simulink model "Nonlinear_Simulink"  (R2025b)
settings: Solver=VariableStepAuto  StartTime=0.0  StopTime=10.0  RelTol=1e-3
undefined symbols (not defined in the file or in its folder): p
settings Model: Creator=chako  LastModifiedBy=emma

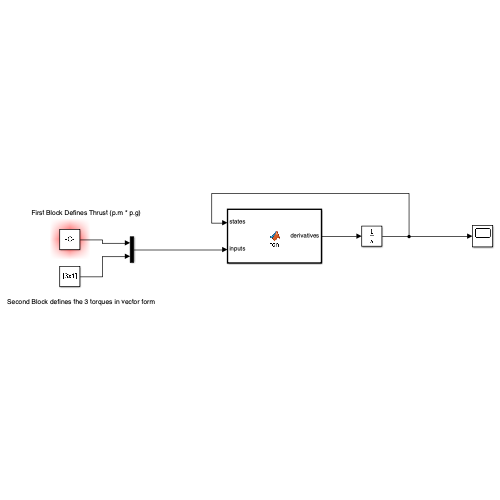
[thumbnail: Simulink's stored preview of the top-level diagram]
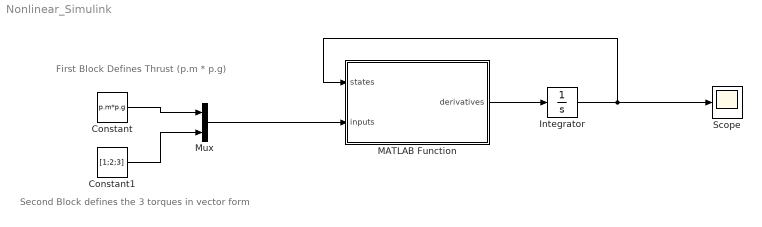
== system Nonlinear_Simulink ==
  note: First Block Defines Thrust (p.m * p.g)
  note: Second Block defines the 3 torques in vector form
  Constant : Constant  Value=p.m*p.g
  Constant1 : Constant  Value=[1;2;3]
  Integrator : Integrator
  MATLAB Function : MATLAB Function  TreatAsAtomicUnit=on
  Mux : Mux  Inputs=2
  Scope : Scope
  wires:
  MATLAB Function/1(derivatives) -> Integrator/1
  Integrator/1 -> MATLAB Function/1(states), Scope/1
  Mux/1 -> MATLAB Function/2(inputs)
  Constant/1 -> Mux/1
  Constant1/1 -> Mux/2

== matlab function Nonlinear_Simulink/MATLAB Function ==
  data: states input size=12; derivatives output size=12; inputs input size=4; parameters parameter
function derivatives = fcn(states, inputs, parameters)

 % I is the inertia matrix
    I = [p.Ixx 0 0;
         0 p.Iyy 0;
         0 0 p.Izz];

    xi= states(1:3); % x, y, z
    xid = states(4:6); %x_prime, y_prime, z_prime
    eta = states(7:9); % roll, pitch, yaw
    etad = states(10:12); % roll_prime, pitch_prime, yaw_prime

    % Cosines of each
    c_roll = cos(eta(1));
    c_pitch = cos(eta(2));
    c_yaw = cos(eta(3));

    % Sines of each
    s_roll = sin(eta(1));
    s_pitch = sin(eta(2));
    s_yaw = sin(eta(3));


    % Derivative of xi is xid

    % Calculative derivatives of xid
    xidd = [0;0;-p.g] - (p.kD/p.m)*xid + ...
        [s_roll*s_yaw + c_roll*s_pitch*c_yaw;
         c_roll*s_pitch*s_yaw - s_roll*c_yaw;
         c_roll*c_pitch]*inputs(1);


    % Derivative of eta is etad
    % Calculative derivatives of etad


    % eta is [phi, theta, psi] = roll pitch yaw
    W = [1  0       -s_pitch;
         0  c_roll  s_phi * c_pitch;
         0 -s_roll  c_roll * c_pitch];
    % v is rpy in body frame
    
    tau_body = [inputs(2);
                inputs(3);
                inputs(4)];
    v = W * etad;
    vd = inv(I) * (tau_body + [(p.Iyy - Izz)*v(2)*v(3); ... 
                               (p.Izz - Ixx)*v(1)*v(3);
                               (p.Ixx - Iyy)*v(1)*v(2)]);
    Wd = [0        0                  -etad(2)*cos(-etad(2));
          0 -etad(1)*s_roll            etad(1)*c_roll*c_pitch;
          0 -etad(1)*c_roll -etad(roll)*s_roll*c_pitch-etad(2)*c_roll*s_pitch];
    etadd = inv(W) * (vd - Wd*etad);
    derivatives = [xid; xidd; etad; etadd];
end
